simulink model "main"  (R2024b)
settings: Solver=VariableStepAuto  StartTime=0.0  StopTime=1.0  RelTol=1e-3
settings Model: Creator=nakamura  LastModifiedBy=nakamura

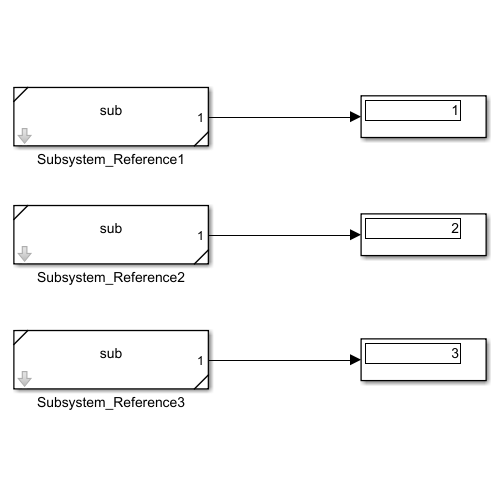
[thumbnail: Simulink's stored preview of the top-level diagram]
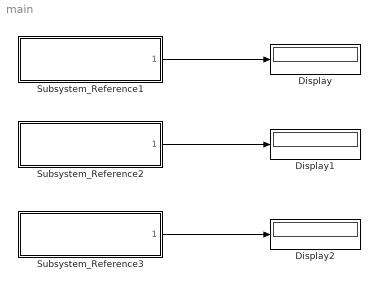
== system main ==
  Display : Display
  Display1 : Display
  Display2 : Display
  Subsystem_Reference1 : Subsystem  ReferencedSubsystem=sub
  Subsystem_Reference2 : Subsystem  ReferencedSubsystem=sub
  Subsystem_Reference3 : Subsystem  ReferencedSubsystem=sub
  wires:
  Subsystem_Reference1/1 -> Display/1
  Subsystem_Reference2/1 -> Display1/1
  Subsystem_Reference3/1 -> Display2/1
